simulink model "diff_mobile_model"  (R2015b)
settings: Solver=VariableStepAuto  StartTime=0.0  StopTime=inf  FixedStep=0.0001  RelTol=1e-3
undefined symbols (not defined in the file): B, Jm, Kt, L, R
settings Model: Creator=root  LastModifiedBy=root

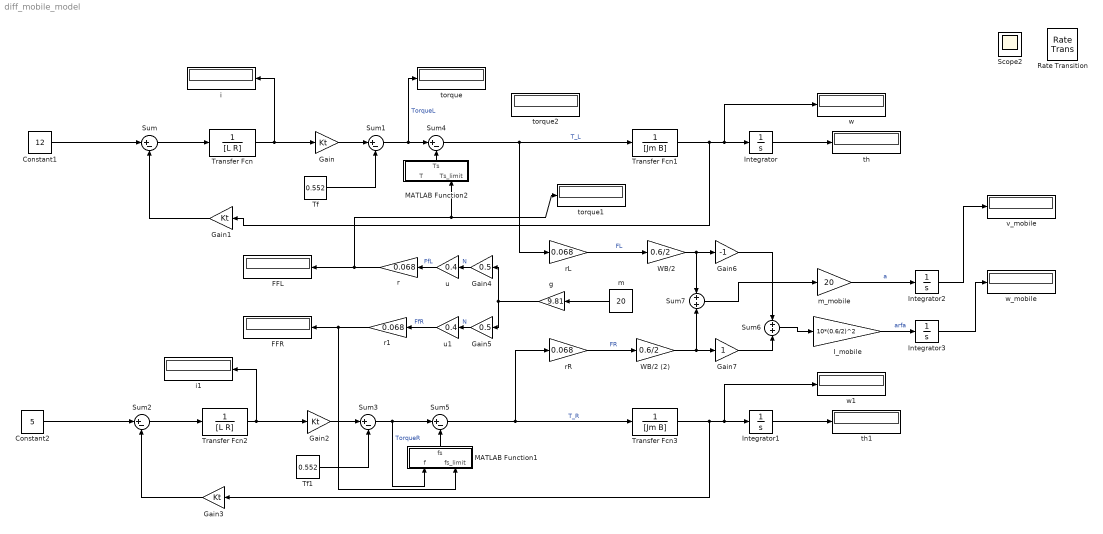
== system diff_mobile_model ==
  Constant1 : Constant  Value=12
  Constant2 : Constant  Value=5
  FFL : Display
  FFR : Display
  Gain{,1..3} (4 alike) : Gain  Gain=Kt
  Gain4 : Gain  Gain=0.5
  Gain5 : Gain  Gain=0.5
  Gain6 : Gain  Gain=-1
  Gain7 : Gain
  I_mobile : Gain  Gain=10*(0.6/2)^2
  Integrator{,1..3} (4 alike) : Integrator
  MATLAB Function1 : MATLAB Function  TreatAsAtomicUnit=on
  MATLAB Function2 : MATLAB Function  TreatAsAtomicUnit=on
  Rate Transition : RateTransition
  Scope2 : Scope
  Sum{,1..5} (6 alike) : Sum  Inputs=|+-
  Sum6 : Sum  Inputs=+|+
  Sum7 : Sum  Inputs=+|+
  Tf : Constant  Value=0.552
  Tf1 : Constant  Value=0.552
  Transfer Fcn : TransferFcn  Denominator=[L R]
  Transfer Fcn1 : TransferFcn  Denominator=[Jm B]
  Transfer Fcn2 : TransferFcn  Denominator=[L R]
  Transfer Fcn3 : TransferFcn  Denominator=[Jm B]
  WB/2 : Gain  Gain=0.6/2
  WB/2 (2) : Gain  Gain=0.6/2
  g : Gain  Gain=9.81
  i : Display
  i1 : Display
  m : Constant  Value=20
  m_mobile : Gain  Gain=20
  r : Gain  Gain=0.068
  r1 : Gain  Gain=0.068
  rL : Gain  Gain=0.068
  rR : Gain  Gain=0.068
  th : Display
  th1 : Display
  torque : Display
  torque1 : Display
  torque2 : Display
  u : Gain  Gain=0.4
  u1 : Gain  Gain=0.4
  v_mobile : Display
  w : Display
  w1 : Display
  w_mobile : Display
  wires:
  Sum/1 -> Transfer Fcn/1
  Gain1/1 -> Sum/2
  Transfer Fcn/1 -> Gain/1, i/1
  Tf/1 -> Sum1/2
  Sum4/1 -> rL/1, Transfer Fcn1/1  "T_L"
  Gain/1 -> Sum1/1
  Constant1/1 -> Sum/1
  Integrator/1 -> th/1
  Transfer Fcn1/1 -> w/1, Integrator/1, Gain1/1
  Sum2/1 -> Transfer Fcn2/1
  Gain3/1 -> Sum2/2
  Transfer Fcn2/1 -> i1/1, Gain2/1
  Sum5/1 -> rR/1, Transfer Fcn3/1  "T_R"
  Gain2/1 -> Sum3/1
  Constant2/1 -> Sum2/1
  Integrator1/1 -> th1/1
  Transfer Fcn3/1 -> Gain3/1, Integrator1/1, w1/1
  Tf1/1 -> Sum3/2
  m/1 -> g/1
  g/1 -> Gain5/1, Gain4/1
  Gain4/1 -> u/1  "N"
  Gain5/1 -> u1/1  "N"
  u/1 -> r/1  "FfL"
  u1/1 -> r1/1  "FfR"
  rL/1 -> WB/2/1  "FL"
  rR/1 -> WB/2 (2)/1  "FR"
  WB/2/1 -> Gain6/1, Sum7/1
  WB/2 (2)/1 -> Sum7/2, Gain7/1
  Gain6/1 -> Sum6/1
  Gain7/1 -> Sum6/2
  Sum6/1 -> I_mobile/1
  Sum7/1 -> m_mobile/1
  m_mobile/1 -> Integrator2/1  "a"
  I_mobile/1 -> Integrator3/1  "arfa"
  Integrator2/1 -> v_mobile/1
  Integrator3/1 -> w_mobile/1
  Sum1/1 -> torque/1, Sum4/1  "TorqueL"
  MATLAB Function1/1(fs) -> Sum5/2
  Sum3/1 -> MATLAB Function1/1(f), Sum5/1  "TorqueR"
  r/1 -> MATLAB Function2/2(Ts_limit), torque1/1, FFL/1
  r1/1 -> MATLAB Function1/2(fs_limit), FFR/1
  MATLAB Function2/1(Ts) -> Sum4/2

== matlab function diff_mobile_model/MATLAB Function1 ==
  data: f input; fs_limit input; fs output
function fs = fcn(f,fs_limit)
%#codegen

if f<=fs_limit
    fs=f;
else
    fs=fs_limit;
end

== matlab function diff_mobile_model/MATLAB Function2 ==
  data: T input; Ts_limit input; Ts output
function Ts = fcn(T,Ts_limit)
%#codegen

if T<=Ts_limit
    Ts=T;
else
    Ts=Ts_limit;
end
